simulink model "BaseFahrzeug"  (Simulink 4.00)
settings: Solver=ode45  StartTime=0.0  StopTime=1180  RelTol=1e-3
values from neighbouring files (symbols this model uses):
  Mp = [-17.8883864542 -0.00131103123218 -0.00197447771532 -0.00115951818457 -0.000680810840922 -0.000399737947721 -0.000234706067872 -0.000137807632584 -8.09137315052e-05 -4.75084869187e-05 -2.78946018106e-05 -1.63783116669e-05 ... (200 elements, 1x200)]    [MondemoECETraj.mat]    (also in MondemoTraj.mat = [-17.8883864542 -0.00131103123218 -0.00197447771532 -0.00115; NeueTraj.m = [Mp V])
  Pload = 200    [DP3.m]    (also in DP4.m; DP5.m)
  Revs = [700 689.515355333 678.827403088 667.93220093 656.825730082 648.204826952 643.716752939 643.137196006 646.288351338 652.783436929 659.590754061 665.368089842 ... (118001 elements, 118001x1)]    [MondemoECETraj.mat]    (also in MondemoTraj.mat; NeueTraj.m = [Revs;V])
  Zeit = [0 0.01 0.02 0.03 0.04 0.05 0.06 0.07 0.08 0.09 0.1 0.11 ... (118001 elements, 118001x1)]    [MondemoECETraj.mat]    (also in MondemoTraj.mat; dp.m = [0:Rows-1]'; dp1.m = [0:Rows-1]'; dp2.m = [0:Rows-1]')
undefined symbols (not defined in the file or in its folder): eng_gen_ratio, gen_effmap_Pels, gen_effmap_speeds, gen_effmap_table, TimeVektor

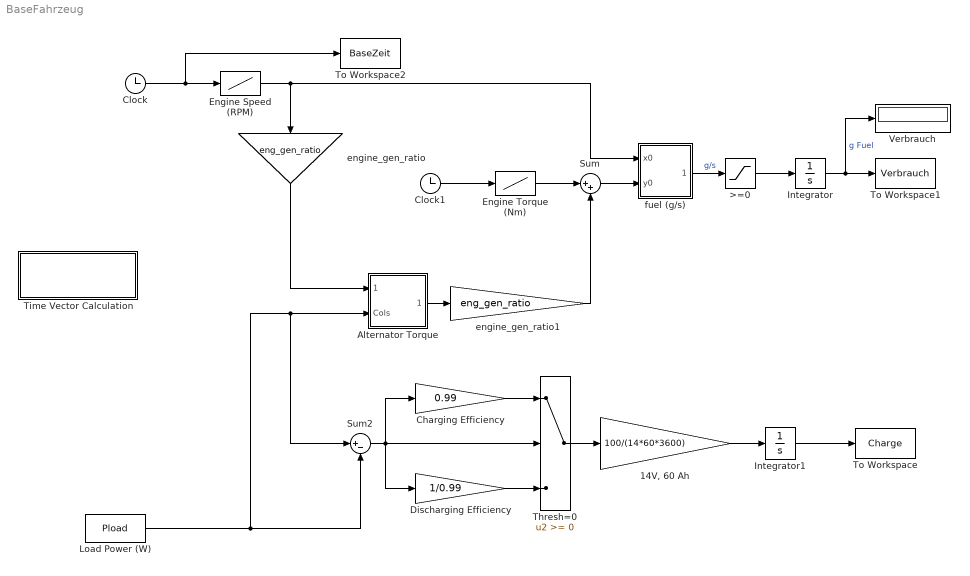
== system BaseFahrzeug ==
  "14V, 60 Ah" : Gain  Gain=100/(14*60*3600)  Multiplication=Element-wise(K.*u)  SaturateOnIntegerOverflow=on
  >=0 : Saturate  UpperLimit=inf  LowerLimit=0  LinearizeAsGain=on
  Alternator Torque : Subsystem  AncestorBlock=|  mask(Lookup Table (2-D)){x=gen_effmap_speeds*30/pi, y=gen_effmap_Pels, t=gen_effmap_table}
      | simulink3/Functions
      | & Tables/Look-Up
      | Table (2-D)
      mask prompts: x "Row:"; y "Column:"; t "Table:"
      mask help: Performs 2-D linear interpolation of input values using the specified input/output table. Extrapolation is performed outside the table boundaries. The first dimension corresponds to the top (or left) input port.
      mask init:
      | [r,c]=size(t);
      | xt=reshape(x,prod(size(x)),1);
      | xi=xt(:,ones(1,c));
      | minx=min(x); maxx=max(x);
      | mint=min(min(t)); maxt=max(max(t));
      settings: RTWFcnNameOpts=Auto  RTWFileNameOpts=Auto
      mask Display: plot(double(xi),double(t),double([minx maxx]),double([mint mint]),double([minx minx]),double([mint maxt]))
  Charging Efficiency : Gain  Gain=0.99  Multiplication=Element-wise(K.*u)  SaturateOnIntegerOverflow=on
  Clock : Clock
      settings: DisplayTime=off  Decimation=10
  Clock1 : Clock
      settings: DisplayTime=off  Decimation=10
  Discharging Efficiency : Gain  Gain=1/0.99  Multiplication=Element-wise(K.*u)  SaturateOnIntegerOverflow=on
  Engine Speed (RPM) : Lookup  InputValues=Zeit  OutputValues=Revs
  Engine Torque (Nm) : Lookup  InputValues=TimeVektor  OutputValues=Mp
  Integrator : Integrator  ExternalReset=none  InitialConditionSource=internal  InitialCondition=0  LimitOutput=off  UpperSaturationLimit=inf  LowerSaturationLimit=-inf  ShowSaturationPort=off  ShowStatePort=off  AbsoluteTolerance=auto
  Integrator1 : Integrator  ExternalReset=none  InitialConditionSource=internal  InitialCondition=0  LimitOutput=off  UpperSaturationLimit=inf  LowerSaturationLimit=-inf  ShowSaturationPort=off  ShowStatePort=off  AbsoluteTolerance=auto
  Load Power (W) : Constant  Value=Pload
  Sum : Sum  Inputs=|++  SaturateOnIntegerOverflow=on
  Sum2 : Sum  Inputs=|+-  SaturateOnIntegerOverflow=on
  Thresh=0 : Switch  Threshold=0
  Time Vector Calculation : Subsystem
      settings: OpenFcn=TimeVektor=[0:N-1];  RTWFcnNameOpts=Auto  RTWFileNameOpts=Auto
  To Workspace : ToWorkspace  VariableName=Charge  SampleTime=-1  SaveFormat=Array
  To Workspace1 : ToWorkspace  VariableName=Verbrauch  SampleTime=-1  SaveFormat=Array
  To Workspace2 : ToWorkspace  VariableName=BaseZeit  SampleTime=-1  SaveFormat=Array
  Verbrauch : Display
      settings: Format=short
  engine_gen_ratio : Gain  Orientation=down  Gain=eng_gen_ratio  Multiplication=Element-wise(K.*u)  SaturateOnIntegerOverflow=on
  engine_gen_ratio1 : Gain  Gain=eng_gen_ratio  Multiplication=Element-wise(K.*u)  SaturateOnIntegerOverflow=on
  fuel (g/s) : Subsystem  mask(2-D Table Lookup){@1=fc_map_spd*fc_spd_scale*30/pi, @2=fc_map_trq*fc_trq_scale, @3=fc_fuel_map*fc_spd_scale*fc_trq_scale}
      mask prompts: @1 "X Index"; @2 "Y Index"; @3 "Table"
      mask help:
      | Two Dimensional Table Lookup
      | The first input corresponds to X Index and the second input corresponds to the Y Index
      mask init:
      | xindex=@1; yindex=@2; table=@3; sftab2chk(xindex,yindex,table);
      settings: RTWFcnNameOpts=Auto  RTWFileNameOpts=Auto
      mask Help: This block returns a linearly interpolated intersection from the table using the X index (which corresponds to the rows of the table) and the Y index (which corresponds to the columns of the table).  Extrapolation is used.
      mask Display: plot(-10,-10,110,110,[90,50,10],[90,40,30],[90,50,10],[50,26,20],[90,50,10],[22,13,10])
  wires:
  Sum/1 -> fuel (g/s)/2(y0)
  Integrator/1 -> To Workspace1/1, Verbrauch/1  "g Fuel"
  fuel (g/s)/1(table out) -> >=0/1  "g/s"
  >=0/1 -> Integrator/1
  Clock/1 -> Engine Speed (RPM)/1, To Workspace2/1
  Engine Speed (RPM)/1 -> fuel (g/s)/1(x0), engine_gen_ratio/1
  Alternator Torque/1(Out1) -> engine_gen_ratio1/1
  engine_gen_ratio/1 -> Alternator Torque/1(Rows)
  engine_gen_ratio1/1 -> Sum/2
  Load Power (W)/1 -> Sum2/2, Alternator Torque/2(Cols), Sum2/1
  Charging Efficiency/1 -> Thresh=0/1
  Sum2/1 -> Charging Efficiency/1, Thresh=0/2, Discharging Efficiency/1
  Discharging Efficiency/1 -> Thresh=0/3
  Thresh=0/1 -> "14V, 60 Ah"/1
  "14V, 60 Ah"/1 -> Integrator1/1
  Integrator1/1 -> To Workspace/1
  Engine Torque (Nm)/1 -> Sum/1
  Clock1/1 -> Engine Torque (Nm)/1

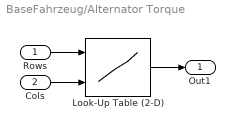
== system BaseFahrzeug/Alternator Torque ==
  Rows : Inport  Port=1  LatchInput=off
  Cols : Inport  Port=2  LatchInput=off
  Look-Up Table (2-D) : Lookup2D  RowIndex=x  ColumnIndex=y  OutputValues=t
  Out1 : Outport  Port=1
  wires:
  Rows/1 -> Look-Up Table (2-D)/1
  Cols/1 -> Look-Up Table (2-D)/2
  Look-Up Table (2-D)/1 -> Out1/1

== system BaseFahrzeug/Time Vector Calculation ==

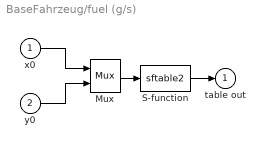
== system BaseFahrzeug/fuel (g/s) ==
  x0 : Inport  Port=1  LatchInput=off
  y0 : Inport  Port=2  LatchInput=off
  Mux : Mux  Inputs=2
      settings: DisplayOption=none
  S-function : S-Function  FunctionName=sftable2  Parameters=xindex, yindex, table  PortCounts=[]  SFunctionModules=''
  table out : Outport  Port=1  InitialOutput=0
  wires:
  Mux/1 -> S-function/1
  x0/1 -> Mux/1
  S-function/1 -> table out/1
  y0/1 -> Mux/2
